simulink model "output"  (R2025a)
settings: Solver=VariableStepAuto  StartTime=0.0  StopTime=10.0  RelTol=1e-3
settings Model: Creator=dinhnamnguyen  LastModifiedBy=dinhnamnguyen

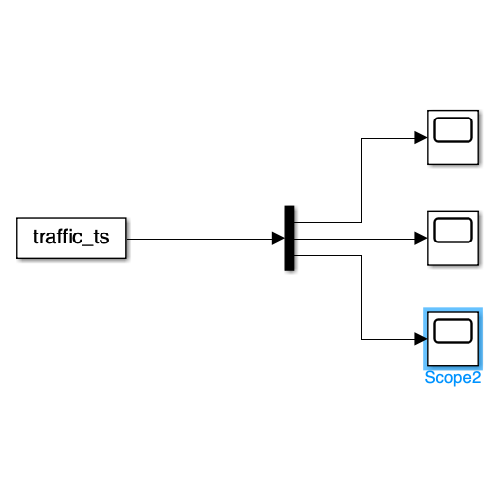
[thumbnail: Simulink's stored preview of the top-level diagram]
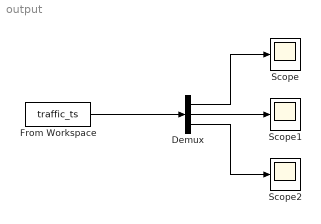
== system output ==
  Demux : Demux  Outputs=3
  From Workspace : FromWorkspace  VariableName=traffic_ts
  Scope : Scope
      settings: ActiveDisplayYMinimum=6.75  ActiveDisplayYMaximum=19.25
  Scope1 : Scope
      settings: ActiveDisplayYMinimum=-0.62499999999999989  ActiveDisplayYMaximum=5.625
  Scope2 : Scope
      settings: ActiveDisplayYMinimum=-1.375  ActiveDisplayYMaximum=2.375  DataLoggingVariableName=ScopeData2
  wires:
  From Workspace/1 -> Demux/1
  Demux/1 -> Scope/1
  Demux/2 -> Scope1/1
  Demux/3 -> Scope2/1
